simulink model "Sim_Kalman_propopject3"  (R2022b)
settings: Solver=VariableStepAuto  StartTime=0.0  StopTime=25  RelTol=1e-3
values from neighbouring files (symbols this model uses):
  A = -jacobian(eqs, xdot) \ jacobian(eqs, x)    [Sim_Init.m]
  Ad = expm(A*Ts)    [Sim_Init.m]
  B = repl(Bm)    [Sim_Init.m]
  Bd = double(Bd)    [Sim_Init.m]
  C1 = repl(C1)    [Sim_Init.m]
  D1 = repl(D1)    [Sim_Init.m]
  Ts = 1e-3    (= 0.001)    [Sim_Init.m]
undefined symbols (not defined in the file or in its folder): Continuous, idss, k1, k_lq, newKi, Rm_kalman, Time
libraries: dspsrcs4 x2, ctrlSharedLib x1
settings Model: Creator=abdul  LastModifiedBy=abdul

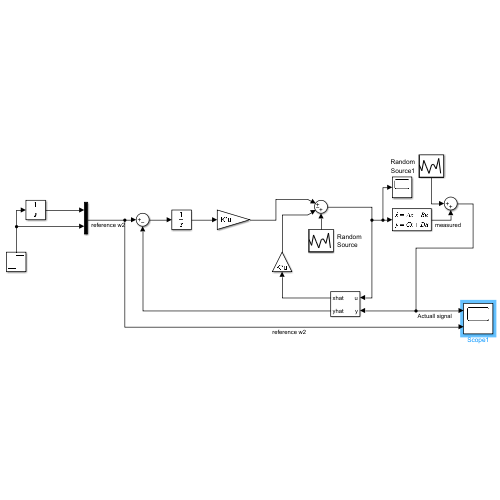
[thumbnail: Simulink's stored preview of the top-level diagram]
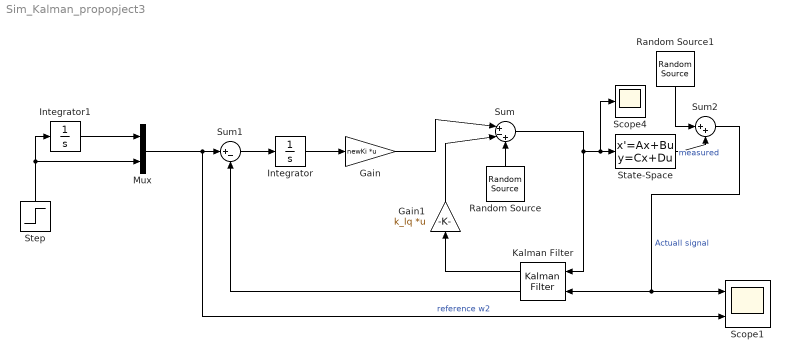
== system Sim_Kalman_propopject3 ==
  Gain : Gain  Gain=newKi  Multiplication=Matrix(K*u)
  Gain1 : Gain  Gain=k_lq  Multiplication=Matrix(K*u)
  Integrator : Integrator
  Integrator1 : Integrator
  Kalman Filter : ctrlSharedLib/Kalman Filter  TimeDomain=Continuous-Time  UseCurrentEstimator=on  ModelSource=Individual A, B, C, D matrices  ModelSourceVariable=idss(Ad,Bd,C1,D1,k1,Ts)  A=A  B=B  C=C1  D=D1  NumberOfStates=1  NumberOfInputs=1  NumberOfOutputs=1  InitialEstimateSource=Dialog  X0=0  P0=10  UseK=off  UseGH=off  NumberOfProcessNoiseInputs=1  G=1  TimeInvariantG=on  H=0  TimeInvariantH=on  Q=Qm_kalman  TimeInvariantQ=on  R=Rm_kalman  TimeInvariantR=on  N=0  TimeInvariantN=on  AddInputPort=on  AddEnablePort=off  OutputEstimatedY=on  OutputP=off  Ts=-1
  Mux : Mux  Inputs=2
  Random Source : dspsrcs4/Random Source  SrcType=Gaussian  NormMethod=Ziggurat  CltLength=12  MinVal=0  MaxVal=1  MeanVal=0  VarVal=1  RepMode=Not repeatable  rawSeed=1  IsInherit=off  SampMode=Discrete  SampTime=1  SampFrame=1  DataType=Double  OutComplex=Real  OutputFrames=off
  Random Source1 : dspsrcs4/Random Source  SrcType=Gaussian  NormMethod=Ziggurat  CltLength=12  MinVal=0  MaxVal=1  MeanVal=0  VarVal=1  RepMode=Not repeatable  rawSeed=1  IsInherit=off  SampMode=Discrete  SampTime=Ts  SampFrame=1  DataType=Double  OutComplex=Real  OutputFrames=off
  Scope1 : Scope  NumInputPorts=2
  Scope4 : Scope
  State-Space : StateSpace  A=A  B=B  C=C1  D=D1  InitialCondition=0
  Step : Step  Before=10  After=100  SampleTime=0
  Sum : Sum  Inputs=|+-+
  Sum1 : Sum  Inputs=|+-
  Sum2 : Sum  Inputs=|++
  wires:
  Sum/1 -> Kalman Filter/1, Scope4/1, State-Space/1
  Step/1 -> Integrator1/1, Mux/2
  Integrator1/1 -> Mux/1
  Gain1/1 -> Sum/2
  Kalman Filter/1 -> Gain1/1
  Gain/1 -> Sum/1
  Kalman Filter/2 -> Sum1/2
  Mux/1 -> Scope1/2, Sum1/1  "reference w2"
  Sum1/1 -> Integrator/1
  Integrator/1 -> Gain/1
  Random Source/1 -> Sum/3
  Random Source1/1 -> Sum2/1
  State-Space/1 -> Sum2/2  "measured"
  Sum2/1 -> Kalman Filter/2, Scope1/1  "Actuall signal"
